simulink model "feedback"  (Simulink 8.3)
settings: Solver=ode113  StartTime=0.0  StopTime=t_end  RelTol=1e-3
values from neighbouring files (symbols this model uses):
  a = 24/t_end    (= 0.4)    [constants.m]
  c_t = 150    [constants.m]
  k_i = 100    [constants.m]
  k_p = 500    [constants.m]
  m_t = 1000    [constants.m]
  r_bar = 50/3600*1000    (= 13.8888888889)    [constants.m]
  v_0 = 10/3600*1000    (= 2.77777777778)    [constants.m]
settings Model: Creator=jamesforbes  LastModifiedBy=Forbesrj
settings OptimizationCC: ExpressionDepthLimit=2147483647
settings DebuggingCC: SolverPrmCheckMsg=none  FcnCallInpInsideContextMsg=EnableAllAsWarning
settings GRTTargetCC: CombineOutputUpdateFcns=on  GRTInterface=off

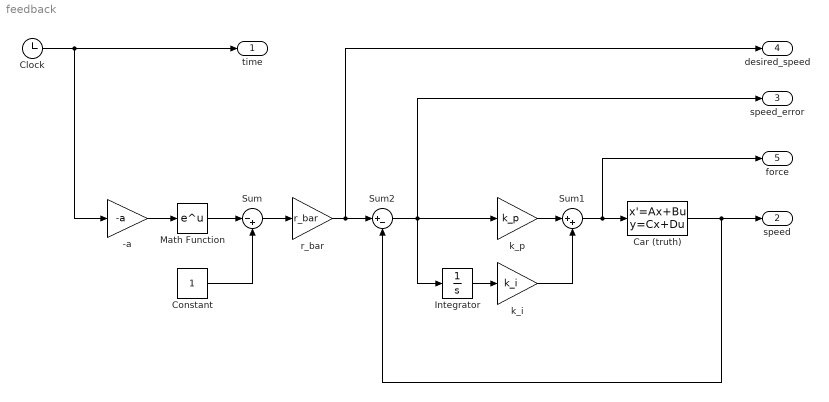
== system feedback ==
  "-a " : Gain  Gain=-a
  Car (truth) : StateSpace  A=-(c_t/m_t)  B=1/m_t  D=0  X0=v_0
  Clock : Clock
  Constant : Constant
  Integrator : Integrator
  Math Function : Math  SaturateOnIntegerOverflow=on
  Sum : Sum  Inputs=|-+
  Sum1 : Sum  Inputs=|++
  Sum2 : Sum  Inputs=|+-
  "k_i " : Gain  Gain=k_i
  k_p : Gain  Gain=k_p
  "r_bar " : Gain  Gain=r_bar
  "time " : Outport
  "speed " : Outport  Port=2
  "speed_error " : Outport  Port=3
  desired_speed : Outport  Port=4
  force : Outport  Port=5
  wires:
  Car (truth)/1 -> "speed "/1, Sum2/2
  Math Function/1 -> Sum/1
  Constant/1 -> Sum/2
  Sum/1 -> "r_bar "/1
  Clock/1 -> "-a "/1, "time "/1
  "-a "/1 -> Math Function/1
  Sum2/1 -> "speed_error "/1, Integrator/1, k_p/1
  "r_bar "/1 -> desired_speed/1, Sum2/1
  Integrator/1 -> "k_i "/1
  Sum1/1 -> force/1, Car (truth)/1
  k_p/1 -> Sum1/1
  "k_i "/1 -> Sum1/2
